simulink model "beetleBotFull"  (R2016a)
settings: Solver=VariableStepAuto  StartTime=0.0  StopTime=simTime  MaxStep=0.001  RelTol=1e-3
model workspace: external: MAT-File C:\Users\dpied\Documents\Carnegie Mellon\2nd Semester\KDC\Project\Segway_Simulation\beetleBot_DataFile.mat (data not in the file)
undefined symbols (not defined in the file or in its folder): Ddecouple, ground_y, Kbalance, Kflight, Kturn, motorSaturation, smiData, state_desired, table, table_height, table_y, X, Y, Z
libraries: sm_lib x149, nesl_utility x15, Contact_Forces_Lib x8, simulink x2
(part 1 of 4)
settings Model: Creator=dpied  LastModifiedBy=dpied
settings GRTTargetCC: GeneratePreprocessorConditionals=Use local settings

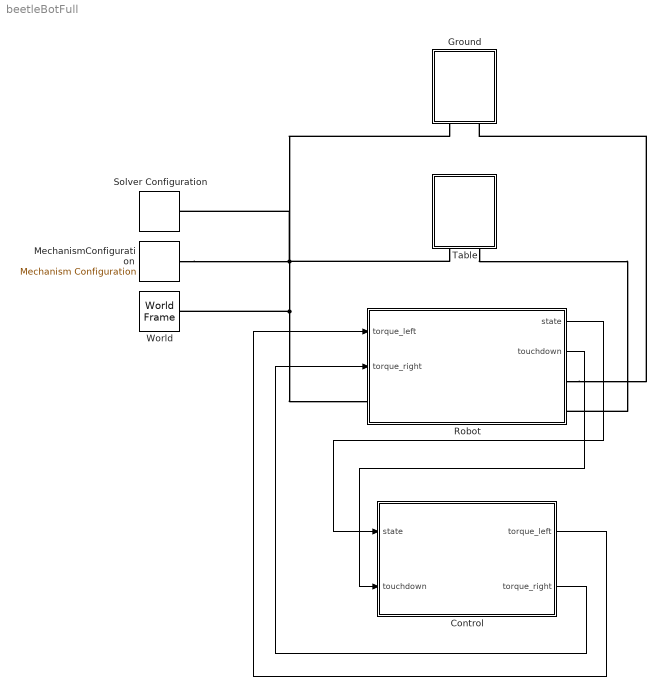
== system beetleBotFull ==
  Control : Subsystem
  Ground : Subsystem
  MechanismConfiguration : sm_lib/Utilities/Mechanism Configuration  UniformGravity=Constant  GravityVector=[0 0 -9.81]  GravityUnits=m/s^2  LinearizationDelta=0.001
  Robot : Subsystem
  Solver Configuration : nesl_utility/Solver Configuration  PhysicalDomain=network_engine_domain  SubClassName=solver  LeftPortType=input  RightPortType=generic  Accelerate=off  Tones=[]  Harmonics=[]  SimulateNoise=off  Profile=off  UseLocalSampling=off  EnableSwitchedLinearOptims=on  FrequencyDomain=off  UseCCode=off  RelTol=0.001  AbsTol=1e-06  MinStep=1e-09  ToWorkspace=off  RevertToSquareIcSolve=off  NumHomotopyIterations=100  PhasorMode=off  PhasorModeNumHarmonics=1  OverrideAbsTol=off  DoDC=off  ResidualTolerance=1e-09  UseLocalSolver=off  LocalSolverChoice=NE_BACKWARD_EULER_ADVANCER  LocalSolverSampleTime=0.001  DoFixedCost=off  MaxNonlinIter=3  MaxModeIter=2  LinearAlgebra=Sparse  DelaysMemoryBudget=1024  AutomaticFiltering=on  FilteringTimeConstant=0.001
  Table : Subsystem
  World : sm_lib/Frames and Transforms/World Frame
  wires:
  Robot/1(state) -> Control/1(state)
  Control/1(torque_left) -> Robot/1(torque_left)
  Control/2(torque_right) -> Robot/2(torque_right)
  Robot/2(touchdown) -> Control/2(touchdown)
  connections:
  MechanismConfiguration/RConn1 -- Robot/LConn1 -- World/RConn1 -- Table/LConn1 -- Ground/LConn1 -- Solver Configuration/RConn1
  Robot/RConn1 -- Ground/LConn2
  Table/LConn2 -- Robot/RConn2

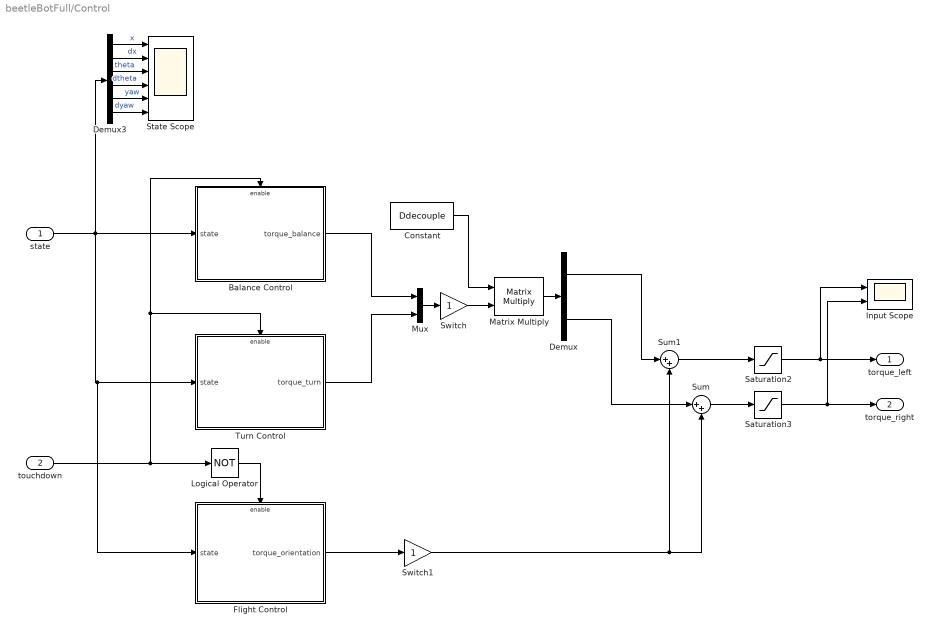
== system beetleBotFull/Control ==
  state : Inport
  touchdown : Inport  Port=2
  Balance Control : Subsystem
  Constant : Constant  Value=Ddecouple
  Demux : Demux  Outputs=2
  Demux3 : Demux  Outputs=6
  Flight Control : Subsystem
  Input Scope : Scope  NumInputPorts=2
  Logical Operator : Logic  Operator=NOT  AllPortsSameDT=off  OutDataTypeStr=boolean
  Matrix Multiply : Product  Multiplication=Matrix(*)
  Mux : Mux  Inputs=2
  Saturation2 : Saturate  UpperLimit=motorSaturation  LowerLimit=-motorSaturation
  Saturation3 : Saturate  UpperLimit=motorSaturation  LowerLimit=-motorSaturation
  State Scope : Scope  NumInputPorts=6
  Sum : Sum  Inputs=|++
  Sum1 : Sum  Inputs=|++
  Switch : Gain
  Switch1 : Gain
  Turn Control : Subsystem
  torque_left : Outport
  torque_right : Outport  Port=2
  wires:
  state/1 -> Flight Control/1(state), Turn Control/1(state), Balance Control/1(state), Demux3/1
  Saturation2/1 -> Input Scope/1, torque_left/1
  Saturation3/1 -> Input Scope/2, torque_right/1
  Demux3/1 -> State Scope/1  "x"
  Demux3/2 -> State Scope/2  "dx"
  touchdown/1 -> Balance Control/Enable, Turn Control/Enable, Logical Operator/1
  Demux3/3 -> State Scope/3  "theta"
  Demux3/4 -> State Scope/4  "dtheta"
  Demux3/5 -> State Scope/5  "yaw"
  Demux3/6 -> State Scope/6  "dyaw"
  Balance Control/1(torque_balance) -> Mux/1
  Turn Control/1(torque_turn) -> Mux/2
  Mux/1 -> Switch/1
  Constant/1 -> Matrix Multiply/1
  Matrix Multiply/1 -> Demux/1
  Switch/1 -> Matrix Multiply/2
  Logical Operator/1 -> Flight Control/Enable
  Sum/1 -> Saturation3/1
  Demux/2 -> Sum/1
  Sum1/1 -> Saturation2/1
  Demux/1 -> Sum1/1
  Flight Control/1(torque_orientation) -> Switch1/1
  Switch1/1 -> Sum1/2, Sum/2

== system beetleBotFull/Ground ==
  Constant : Constant  Value=0
  Constant1 : Constant  Value=0
  Ground : Subsystem  Tag=CustomStyle
  Simulink-PS Converter : nesl_utility/Simulink-PS Converter  PhysicalDomain=network_engine_domain  SubClassName=ps_input  LeftPortType=input  RightPortType=output  PseudoPeriodic=off  Frequencies=[]  NoiseDistribution=none  NoiseParameters=[]  Unit=1  AffineConversion=off  InputFiltering=off  SimscapeFilterOrder=1  InputFilterTimeConstant=0.001  UdotUserProvided=1
  Simulink-PS Converter1 : nesl_utility/Simulink-PS Converter  PhysicalDomain=network_engine_domain  SubClassName=ps_input  LeftPortType=input  RightPortType=output  PseudoPeriodic=off  Frequencies=[]  NoiseDistribution=none  NoiseParameters=[]  Unit=1  AffineConversion=off  InputFiltering=off  SimscapeFilterOrder=1  InputFilterTimeConstant=0.001  UdotUserProvided=1
  Universal Joint : sm_lib/Joints/Universal Joint  SenseConstraintForce=off  SenseConstraintForceX=off  SenseConstraintForceY=off  SenseConstraintForceZ=off  SenseConstraintTorque=off  SenseConstraintTorqueX=off  SenseConstraintTorqueY=off  SenseConstraintTorqueZ=off  SenseTotalForce=off  SenseTotalForceX=off  SenseTotalForceY=off  SenseTotalForceZ=off  SenseTotalTorque=off  SenseTotalTorqueX=off  SenseTotalTorqueY=off  SenseTotalTorqueZ=off  CompositeWrenchDir=FollowerOnBase  CompositeWrenchFrame=BaseFrame  RxEquilibriumPosition=0  RxEquilibriumPositionUnits=deg  RxSpringStiffness=0  RxSpringStiffnessUnits=N*m/deg  RxDampingCoefficient=0  RxDampingCoefficientUnits=N*m/(deg/s)  RxTorqueActuationMode=ComputedTorque  RxMotionActuationMode=InputMotion  RxSensePosition=off  RxSenseVelocity=off  RxSenseAcceleration=off  RxSenseTorqueForce=off  RxPositionTargetSpecify=off  RxPositionTargetPriority=High  RxPositionTargetValue=0  RxPositionTargetValueUnits=deg  RxVelocityTargetSpecify=off  RxVelocityTargetPriority=High  RxVelocityTargetValue=0  RxVelocityTargetValueUnits=deg/s  RyEquilibriumPosition=0  RyEquilibriumPositionUnits=deg  RySpringStiffness=0  RySpringStiffnessUnits=N*m/deg  RyDampingCoefficient=0  RyDampingCoefficientUnits=N*m/(deg/s)  RyTorqueActuationMode=ComputedTorque  RyMotionActuationMode=InputMotion  RySensePosition=off  RySenseVelocity=off  RySenseAcceleration=off  RySenseTorqueForce=off  RyPositionTargetSpecify=off  RyPositionTargetPriority=High  RyPositionTargetValue=0  RyPositionTargetValueUnits=deg  RyVelocityTargetSpecify=off  RyVelocityTargetPriority=High  RyVelocityTargetValue=0  RyVelocityTargetValueUnits=deg/s
  worldFrame : PMIOPort  Port=1  Side=Left
  groundFrame : PMIOPort  Port=2  Side=Left
  wires:
  Constant/1 -> Simulink-PS Converter/1
  Constant1/1 -> Simulink-PS Converter1/1
  connections:
  Ground/LConn1 -- Universal Joint/RConn1
  Simulink-PS Converter/RConn1 -- Universal Joint/LConn2
  Simulink-PS Converter1/RConn1 -- Universal Joint/LConn3
  groundFrame/RConn1 -- Ground/RConn1
  Universal Joint/LConn1 -- worldFrame/RConn1

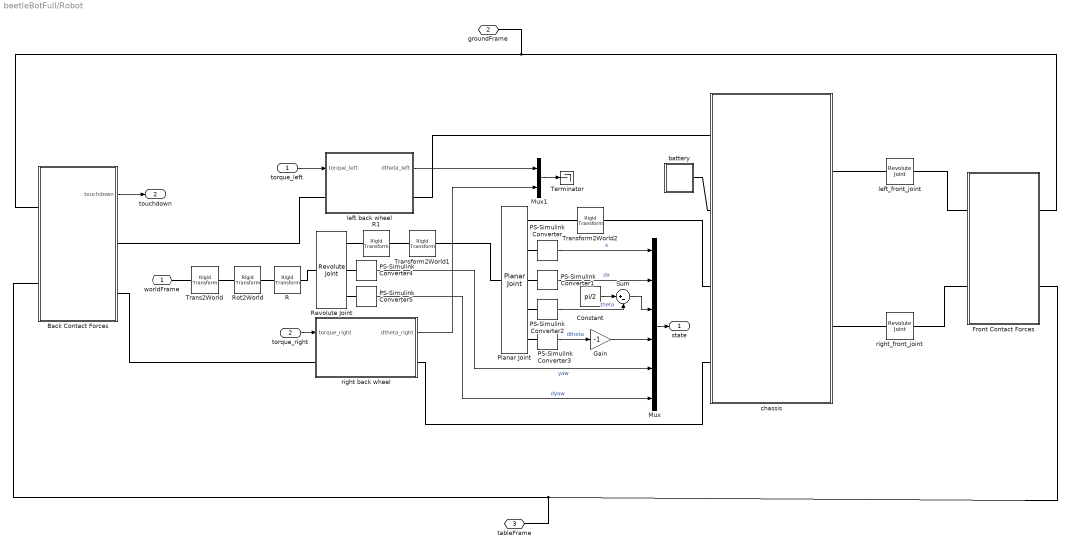
== system beetleBotFull/Robot ==
  torque_left : Inport
  torque_right : Inport  Port=2
  Back Contact Forces : Subsystem
  Constant : Constant  Value=pi/2
  Front Contact Forces : Subsystem
  Gain : Gain  Gain=-1
  Mux : Mux  Inputs=6
  Mux1 : Mux  Inputs=2
  PS-Simulink Converter{,1..5} (6 alike) : nesl_utility/PS-Simulink Converter  PhysicalDomain=network_engine_domain  SubClassName=ps_output  LeftPortType=input  RightPortType=output  PseudoPeriodic=off  Frequencies=[]  Unit=1  AffineConversion=off
  Planar Joint : sm_lib/Joints/Planar Joint  SenseConstraintForce=off  SenseConstraintForceX=off  SenseConstraintForceY=off  SenseConstraintForceZ=off  SenseConstraintTorque=off  SenseConstraintTorqueX=off  SenseConstraintTorqueY=off  SenseConstraintTorqueZ=off  SenseTotalForce=off  SenseTotalForceX=off  SenseTotalForceY=off  SenseTotalForceZ=off  SenseTotalTorque=off  SenseTotalTorqueX=off  SenseTotalTorqueY=off  SenseTotalTorqueZ=off  CompositeWrenchDir=FollowerOnBase  CompositeWrenchFrame=BaseFrame  PxEquilibriumPosition=0  PxEquilibriumPositionUnits=m  PxSpringStiffness=0  PxSpringStiffnessUnits=N/m  PxDampingCoefficient=0  PxDampingCoefficientUnits=N/(m/s)  PxTorqueActuationMode=NoTorque  PxMotionActuationMode=ComputedMotion  PxSensePosition=on  PxSenseVelocity=on  PxSenseAcceleration=off  PxSenseTorqueForce=off  PxPositionTargetSpecify=on  PxPositionTargetPriority=High  PxPositionTargetValue=x_initial  PxPositionTargetValueUnits=m  PxVelocityTargetSpecify=on  PxVelocityTargetPriority=High  PxVelocityTargetValue=dx_initial  PxVelocityTargetValueUnits=m/s  PyEquilibriumPosition=0  PyEquilibriumPositionUnits=m  PySpringStiffness=0  PySpringStiffnessUnits=N/m  PyDampingCoefficient=0  PyDampingCoefficientUnits=N/(m/s)  PyTorqueActuationMode=NoTorque  PyMotionActuationMode=ComputedMotion  PySensePosition=off  PySenseVelocity=off  PySenseAcceleration=off  PySenseTorqueForce=off  PyPositionTargetSpecify=on  PyPositionTargetPriority=High  PyPositionTargetValue=initial_height  PyPositionTargetValueUnits=m  PyVelocityTargetSpecify=off  PyVelocityTargetPriority=High  PyVelocityTargetValue=0  PyVelocityTargetValueUnits=m/s  RzEquilibriumPosition=0  RzEquilibriumPositionUnits=deg  RzSpringStiffness=0  RzSpringStiffnessUnits=N*m/deg  RzDampingCoefficient=0  RzDampingCoefficientUnits=N*m/(deg/s)  RzTorqueActuationMode=NoTorque  RzMotionActuationMode=ComputedMotion  RzSensePosition=on  RzSenseVelocity=on  RzSenseAcceleration=off  RzSenseTorqueForce=off  RzPositionTargetSpecify=on  RzPositionTargetPriority=High  RzPositionTargetValue=theta_initial  RzPositionTargetValueUnits=deg  RzVelocityTargetSpecify=off  RzVelocityTargetPriority=High  RzVelocityTargetValue=0  RzVelocityTargetValueUnits=deg/s
  R : sm_lib/Frames and Transforms/Rigid Transform  TranslationMethod=None  TranslationLengthUnit=mm  TranslationStandardAxis=+Z  TranslationStandardOffset=0  TranslationCartesianOffset=smiData.RigidTransform(51).translation  TranslationROffset=0  TranslationROffsetUnits=m  TranslationZOffset=0  TranslationZOffsetUnits=m  TranslationThetaOffset=0  TranslationThetaOffsetUnits=deg  RotationMethod=StandardAxis  RotationAngleUnits=rad  RotationStandardAxis=+X  RotationAngle=-pi/2  RotationArbitraryAxis=smiData.RigidTransform(51).axis  FollAlignAxisA=+X  BaseAlignAxisA=+Y  FollAlignAxisB=+Y  BaseAlignAxisB=+Z  RotationSequenceAxes=FollowerAxes  RotationSequence=XYX  RotationSequenceAngles=[0 0 0]  RotationSequenceAnglesUnits=deg  RotationMatrix=[1 0 0; 0 1 0; 0 0 1]
  R1 : sm_lib/Frames and Transforms/Rigid Transform  TranslationMethod=None  TranslationLengthUnit=mm  TranslationStandardAxis=+Z  TranslationStandardOffset=0  TranslationCartesianOffset=smiData.RigidTransform(51).translation  TranslationROffset=0  TranslationROffsetUnits=m  TranslationZOffset=0  TranslationZOffsetUnits=m  TranslationThetaOffset=0  TranslationThetaOffsetUnits=deg  RotationMethod=StandardAxis  RotationAngleUnits=rad  RotationStandardAxis=+X  RotationAngle=pi/2  RotationArbitraryAxis=smiData.RigidTransform(51).axis  FollAlignAxisA=+X  BaseAlignAxisA=+Y  FollAlignAxisB=+Y  BaseAlignAxisB=+Z  RotationSequenceAxes=FollowerAxes  RotationSequence=XYX  RotationSequenceAngles=[0 0 0]  RotationSequenceAnglesUnits=deg  RotationMatrix=[1 0 0; 0 1 0; 0 0 1]
  Revolute Joint : sm_lib/Joints/Revolute Joint  SenseConstraintForce=off  SenseConstraintForceX=off  SenseConstraintForceY=off  SenseConstraintForceZ=off  SenseConstraintTorque=off  SenseConstraintTorqueX=off  SenseConstraintTorqueY=off  SenseConstraintTorqueZ=off  SenseTotalForce=off  SenseTotalForceX=off  SenseTotalForceY=off  SenseTotalForceZ=off  SenseTotalTorque=off  SenseTotalTorqueX=off  SenseTotalTorqueY=off  SenseTotalTorqueZ=off  CompositeWrenchDir=FollowerOnBase  CompositeWrenchFrame=BaseFrame  EquilibriumPosition=0  EquilibriumPositionUnits=deg  SpringStiffness=0  SpringStiffnessUnits=N*m/deg  DampingCoefficient=0  DampingCoefficientUnits=N*m/(deg/s)  TorqueActuationMode=NoTorque  MotionActuationMode=ComputedMotion  SensePosition=on  SenseVelocity=on  SenseAcceleration=off  SenseTorqueForce=off  PositionTargetSpecify=off  PositionTargetPriority=High  PositionTargetValue=0  PositionTargetValueUnits=deg  VelocityTargetSpecify=off  VelocityTargetPriority=High  VelocityTargetValue=0  VelocityTargetValueUnits=deg/s
  Rot2World : sm_lib/Frames and Transforms/Rigid Transform  TranslationMethod=None  TranslationLengthUnit=mm  TranslationStandardAxis=+Z  TranslationStandardOffset=0  TranslationCartesianOffset=smiData.RigidTransform(51).translation  TranslationROffset=0  TranslationROffsetUnits=m  TranslationZOffset=0  TranslationZOffsetUnits=m  TranslationThetaOffset=0  TranslationThetaOffsetUnits=deg  RotationMethod=StandardAxis  RotationAngleUnits=rad  RotationStandardAxis=+X  RotationAngle=pi/2  RotationArbitraryAxis=smiData.RigidTransform(51).axis  FollAlignAxisA=+X  BaseAlignAxisA=+Y  FollAlignAxisB=+Y  BaseAlignAxisB=+Z  RotationSequenceAxes=FollowerAxes  RotationSequence=XYX  RotationSequenceAngles=[0 0 0]  RotationSequenceAnglesUnits=deg  RotationMatrix=[1 0 0; 0 1 0; 0 0 1]
  Sum : Sum  Inputs=|+-
  Terminator : Terminator
  Trans2World : sm_lib/Frames and Transforms/Rigid Transform  TranslationMethod=Cartesian  TranslationLengthUnit=m  TranslationStandardAxis=+Z  TranslationStandardOffset=0  TranslationCartesianOffset=[0 0 0.118]  TranslationROffset=0  TranslationROffsetUnits=m  TranslationZOffset=0  TranslationZOffsetUnits=m  TranslationThetaOffset=0  TranslationThetaOffsetUnits=deg  RotationMethod=None  RotationAngleUnits=rad  RotationStandardAxis=+X  RotationAngle=pi/2  RotationArbitraryAxis=smiData.RigidTransform(51).axis  FollAlignAxisA=+X  BaseAlignAxisA=+Y  FollAlignAxisB=+Y  BaseAlignAxisB=+Z  RotationSequenceAxes=FollowerAxes  RotationSequence=XYX  RotationSequenceAngles=[0 0 0]  RotationSequenceAnglesUnits=deg  RotationMatrix=[1 0 0; 0 1 0; 0 0 1]
  Transform2World1 : sm_lib/Frames and Transforms/Rigid Transform  TranslationMethod=None  TranslationLengthUnit=mm  TranslationStandardAxis=+Z  TranslationStandardOffset=0  TranslationCartesianOffset=smiData.RigidTransform(51).translation  TranslationROffset=0  TranslationROffsetUnits=m  TranslationZOffset=0  TranslationZOffsetUnits=m  TranslationThetaOffset=0  TranslationThetaOffsetUnits=deg  RotationMethod=StandardAxis  RotationAngleUnits=rad  RotationStandardAxis=+Y  RotationAngle=-pi/2  RotationArbitraryAxis=smiData.RigidTransform(51).axis  FollAlignAxisA=+X  BaseAlignAxisA=+Y  FollAlignAxisB=+Y  BaseAlignAxisB=+Z  RotationSequenceAxes=FollowerAxes  RotationSequence=XYX  RotationSequenceAngles=[0 0 0]  RotationSequenceAnglesUnits=deg  RotationMatrix=[1 0 0; 0 1 0; 0 0 1]
  Transform2World2 : sm_lib/Frames and Transforms/Rigid Transform  TranslationMethod=None  TranslationLengthUnit=mm  TranslationStandardAxis=+Z  TranslationStandardOffset=0  TranslationCartesianOffset=smiData.RigidTransform(51).translation  TranslationROffset=0  TranslationROffsetUnits=m  TranslationZOffset=0  TranslationZOffsetUnits=m  TranslationThetaOffset=0  TranslationThetaOffsetUnits=deg  RotationMethod=StandardAxis  RotationAngleUnits=rad  RotationStandardAxis=+Y  RotationAngle=pi/2  RotationArbitraryAxis=smiData.RigidTransform(51).axis  FollAlignAxisA=+X  BaseAlignAxisA=+Y  FollAlignAxisB=+Y  BaseAlignAxisB=+Z  RotationSequenceAxes=FollowerAxes  RotationSequence=XYX  RotationSequenceAngles=[0 0 0]  RotationSequenceAnglesUnits=deg  RotationMatrix=[1 0 0; 0 1 0; 0 0 1]
  battery : Subsystem
  chassis : Subsystem
  left back wheel : Subsystem
  left_front_joint : sm_lib/Joints/Revolute Joint  SenseConstraintForce=off  SenseConstraintForceX=off  SenseConstraintForceY=off  SenseConstraintForceZ=off  SenseConstraintTorque=off  SenseConstraintTorqueX=off  SenseConstraintTorqueY=off  SenseConstraintTorqueZ=off  SenseTotalForce=off  SenseTotalForceX=off  SenseTotalForceY=off  SenseTotalForceZ=off  SenseTotalTorque=off  SenseTotalTorqueX=off  SenseTotalTorqueY=off  SenseTotalTorqueZ=off  CompositeWrenchDir=FollowerOnBase  CompositeWrenchFrame=BaseFrame  EquilibriumPosition=0  EquilibriumPositionUnits=rad  SpringStiffness=0  SpringStiffnessUnits=m*N/rad  DampingCoefficient=0  DampingCoefficientUnits=m*s*N/rad  TorqueActuationMode=NoTorque  MotionActuationMode=ComputedMotion  SensePosition=off  SenseVelocity=off  SenseAcceleration=off  SenseTorqueForce=off  PositionTargetSpecify=on  PositionTargetPriority=Low  PositionTargetValue=0  PositionTargetValueUnits=deg  VelocityTargetSpecify=off  VelocityTargetPriority=High  VelocityTargetValue=0  VelocityTargetValueUnits=deg/s
  right back wheel : Subsystem
  right_front_joint : sm_lib/Joints/Revolute Joint  SenseConstraintForce=off  SenseConstraintForceX=off  SenseConstraintForceY=off  SenseConstraintForceZ=off  SenseConstraintTorque=off  SenseConstraintTorqueX=off  SenseConstraintTorqueY=off  SenseConstraintTorqueZ=off  SenseTotalForce=off  SenseTotalForceX=off  SenseTotalForceY=off  SenseTotalForceZ=off  SenseTotalTorque=off  SenseTotalTorqueX=off  SenseTotalTorqueY=off  SenseTotalTorqueZ=off  CompositeWrenchDir=FollowerOnBase  CompositeWrenchFrame=BaseFrame  EquilibriumPosition=0  EquilibriumPositionUnits=rad  SpringStiffness=0  SpringStiffnessUnits=m*N/rad  DampingCoefficient=0  DampingCoefficientUnits=m*s*N/rad  TorqueActuationMode=NoTorque  MotionActuationMode=ComputedMotion  SensePosition=off  SenseVelocity=off  SenseAcceleration=off  SenseTorqueForce=off  PositionTargetSpecify=on  PositionTargetPriority=Low  PositionTargetValue=0  PositionTargetValueUnits=deg  VelocityTargetSpecify=off  VelocityTargetPriority=High  VelocityTargetValue=0  VelocityTargetValueUnits=deg/s
  worldFrame : PMIOPort  Port=1  Side=Left
  groundFrame : PMIOPort  Port=2  Side=Right
  tableFrame : PMIOPort  Port=3  Side=Right
  state : Outport
  touchdown : Outport  Port=2
  wires:
  torque_left/1 -> left back wheel/1(torque_left)
  Mux/1 -> state/1
  Mux1/1 -> Terminator/1
  left back wheel/1(dtheta_left) -> Mux1/1
  right back wheel/1(dtheta_right) -> Mux1/2
  torque_right/1 -> right back wheel/1(torque_right)
  Back Contact Forces/1(touchdown) -> touchdown/1
  PS-Simulink Converter2/1 -> Sum/2  "theta"
  PS-Simulink Converter3/1 -> Gain/1  "dtheta"
  Sum/1 -> Mux/3
  Constant/1 -> Sum/1
  PS-Simulink Converter/1 -> Mux/1  "x"
  PS-Simulink Converter1/1 -> Mux/2  "dx"
  Gain/1 -> Mux/4
  PS-Simulink Converter4/1 -> Mux/5  "yaw"
  PS-Simulink Converter5/1 -> Mux/6  "dyaw"
  connections:
  Trans2World/RConn1 -- Rot2World/LConn1
  battery/LConn1 -- chassis/LConn2
  worldFrame/RConn1 -- Trans2World/LConn1
  chassis/LConn1 -- left back wheel/RConn1
  chassis/LConn4 -- right back wheel/RConn1
  Transform2World2/LConn1 -- Planar Joint/RConn1
  left_front_joint/LConn1 -- chassis/RConn1
  right_front_joint/LConn1 -- chassis/RConn2
  Transform2World2/RConn1 -- chassis/LConn3
  R/LConn1 -- Rot2World/RConn1
  groundFrame/RConn1 -- Back Contact Forces/LConn1 -- Front Contact Forces/RConn1
  Front Contact Forces/LConn1 -- left_front_joint/RConn1
  Front Contact Forces/LConn2 -- right_front_joint/RConn1
  Back Contact Forces/RConn1 -- left back wheel/LConn1
  Back Contact Forces/RConn2 -- right back wheel/LConn1
  PS-Simulink Converter/LConn1 -- Planar Joint/RConn2
  PS-Simulink Converter1/LConn1 -- Planar Joint/RConn3
  Planar Joint/RConn4 -- PS-Simulink Converter2/LConn1
  Planar Joint/RConn5 -- PS-Simulink Converter3/LConn1
  Transform2World1/RConn1 -- Planar Joint/LConn1
  Transform2World1/LConn1 -- R1/RConn1
  Revolute Joint/LConn1 -- R/RConn1
  R1/LConn1 -- Revolute Joint/RConn1
  PS-Simulink Converter4/LConn1 -- Revolute Joint/RConn2
  PS-Simulink Converter5/LConn1 -- Revolute Joint/RConn3
  tableFrame/RConn1 -- Back Contact Forces/LConn2 -- Front Contact Forces/RConn2

== system beetleBotFull/Table ==
  Constant : Constant  Value=0
  Constant1 : Constant  Value=0
  Simulink-PS Converter : nesl_utility/Simulink-PS Converter  PhysicalDomain=network_engine_domain  SubClassName=ps_input  LeftPortType=input  RightPortType=output  PseudoPeriodic=off  Frequencies=[]  NoiseDistribution=none  NoiseParameters=[]  Unit=1  AffineConversion=off  InputFiltering=off  SimscapeFilterOrder=1  InputFilterTimeConstant=0.001  UdotUserProvided=1
  Simulink-PS Converter1 : nesl_utility/Simulink-PS Converter  PhysicalDomain=network_engine_domain  SubClassName=ps_input  LeftPortType=input  RightPortType=output  PseudoPeriodic=off  Frequencies=[]  NoiseDistribution=none  NoiseParameters=[]  Unit=1  AffineConversion=off  InputFiltering=off  SimscapeFilterOrder=1  InputFilterTimeConstant=0.001  UdotUserProvided=1
  Table : Subsystem  Tag=CustomStyle
  Universal Joint : sm_lib/Joints/Universal Joint  SenseConstraintForce=off  SenseConstraintForceX=off  SenseConstraintForceY=off  SenseConstraintForceZ=off  SenseConstraintTorque=off  SenseConstraintTorqueX=off  SenseConstraintTorqueY=off  SenseConstraintTorqueZ=off  SenseTotalForce=off  SenseTotalForceX=off  SenseTotalForceY=off  SenseTotalForceZ=off  SenseTotalTorque=off  SenseTotalTorqueX=off  SenseTotalTorqueY=off  SenseTotalTorqueZ=off  CompositeWrenchDir=FollowerOnBase  CompositeWrenchFrame=BaseFrame  RxEquilibriumPosition=0  RxEquilibriumPositionUnits=deg  RxSpringStiffness=0  RxSpringStiffnessUnits=N*m/deg  RxDampingCoefficient=0  RxDampingCoefficientUnits=N*m/(deg/s)  RxTorqueActuationMode=ComputedTorque  RxMotionActuationMode=InputMotion  RxSensePosition=off  RxSenseVelocity=off  RxSenseAcceleration=off  RxSenseTorqueForce=off  RxPositionTargetSpecify=off  RxPositionTargetPriority=High  RxPositionTargetValue=0  RxPositionTargetValueUnits=deg  RxVelocityTargetSpecify=off  RxVelocityTargetPriority=High  RxVelocityTargetValue=0  RxVelocityTargetValueUnits=deg/s  RyEquilibriumPosition=0  RyEquilibriumPositionUnits=deg  RySpringStiffness=0  RySpringStiffnessUnits=N*m/deg  RyDampingCoefficient=0  RyDampingCoefficientUnits=N*m/(deg/s)  RyTorqueActuationMode=ComputedTorque  RyMotionActuationMode=InputMotion  RySensePosition=off  RySenseVelocity=off  RySenseAcceleration=off  RySenseTorqueForce=off  RyPositionTargetSpecify=off  RyPositionTargetPriority=High  RyPositionTargetValue=0  RyPositionTargetValueUnits=deg  RyVelocityTargetSpecify=off  RyVelocityTargetPriority=High  RyVelocityTargetValue=0  RyVelocityTargetValueUnits=deg/s
  worldFrame : PMIOPort  Port=1  Side=Left
  tableFrame : PMIOPort  Port=2  Side=Left
  wires:
  Constant/1 -> Simulink-PS Converter/1
  Constant1/1 -> Simulink-PS Converter1/1
  connections:
  Table/LConn1 -- Universal Joint/RConn1
  Simulink-PS Converter/RConn1 -- Universal Joint/LConn2
  Simulink-PS Converter1/RConn1 -- Universal Joint/LConn3
  tableFrame/RConn1 -- Table/RConn1
  Universal Joint/LConn1 -- worldFrame/RConn1

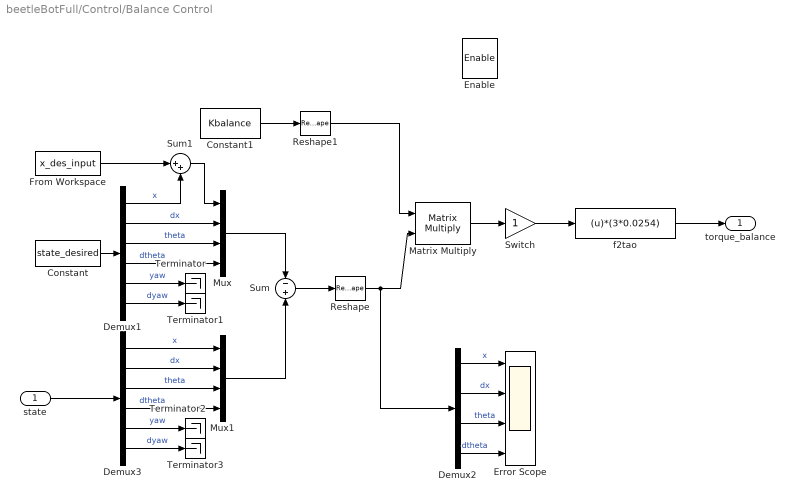
== system beetleBotFull/Control/Balance Control ==
  state : Inport
  Enable : EnablePort
  Constant : Constant  Value=state_desired
  Constant1 : Constant  Value=Kbalance
  Demux1 : Demux  Outputs=6
  Demux2 : Demux
  Demux3 : Demux  Outputs=6
  Error Scope : Scope  NumInputPorts=4
  From Workspace : FromWorkspace  VariableName=x_des_input  SampleTime=0
  Matrix Multiply : Product  Multiplication=Matrix(*)
  Mux : Mux
  Mux1 : Mux
  Reshape : Reshape  OutputDimensionality=Column vector (2-D)
  Reshape1 : Reshape  OutputDimensionality=Row vector (2-D)
  Sum : Sum  Inputs=-+
  Sum1 : Sum  Inputs=|++
  Switch : Gain
  Terminator{,1..3} (4 alike) : Terminator
  f2tao : Fcn  Expr=(u)*(3*0.0254)
  torque_balance : Outport  OutputWhenDisabled=reset  InitialOutput=0
  wires:
  Matrix Multiply/1 -> Switch/1
  Constant1/1 -> Reshape1/1
  Sum/1 -> Reshape/1
  Reshape1/1 -> Matrix Multiply/1
  Switch/1 -> f2tao/1
  Constant/1 -> Demux1/1
  Mux/1 -> Sum/1
  Demux1/1 -> Sum1/2  "x"
  Sum1/1 -> Mux/1
  From Workspace/1 -> Sum1/1
  Demux1/2 -> Mux/2  "dx"
  Demux1/3 -> Mux/3  "theta"
  Demux1/4 -> Mux/4  "dtheta"
  Demux2/1 -> Error Scope/1  "x"
  Demux2/2 -> Error Scope/2  "dx"
  Demux2/3 -> Error Scope/3  "theta"
  Demux2/4 -> Error Scope/4  "dtheta"
  Demux1/5 -> Terminator/1  "yaw"
  Demux1/6 -> Terminator1/1  "dyaw"
  Mux1/1 -> Sum/2
  Demux3/2 -> Mux1/2  "dx"
  Demux3/3 -> Mux1/3  "theta"
  Demux3/4 -> Mux1/4  "dtheta"
  Demux3/5 -> Terminator2/1  "yaw"
  Demux3/6 -> Terminator3/1  "dyaw"
  Demux3/1 -> Mux1/1  "x"
  state/1 -> Demux3/1
  f2tao/1 -> torque_balance/1
  Reshape/1 -> Demux2/1, Matrix Multiply/2

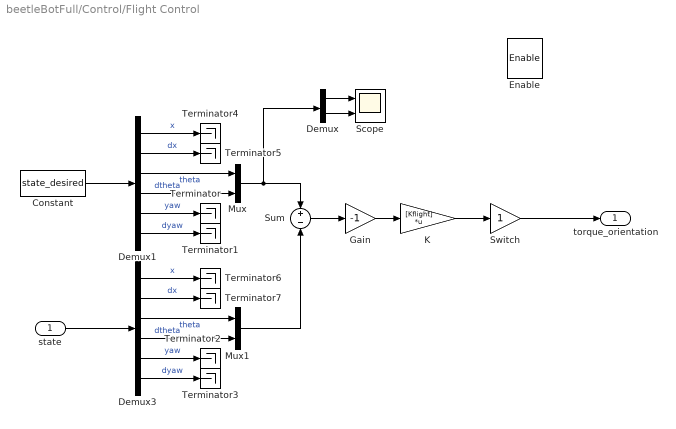
== system beetleBotFull/Control/Flight Control ==
  state : Inport
  Enable : EnablePort
  Constant : Constant  Value=state_desired
  Demux : Demux  Outputs=2
  Demux1 : Demux  Outputs=6
  Demux3 : Demux  Outputs=6
  Gain : Gain  Gain=-1
  K : Gain  Gain=[Kflight]  Multiplication=Matrix(K*u)
  Mux : Mux  Inputs=2
  Mux1 : Mux  Inputs=2
  Scope : Scope  NumInputPorts=2
  Sum : Sum  Inputs=+-
  Switch : Gain
  Terminator{,1..7} (8 alike) : Terminator
  torque_orientation : Outport  OutputWhenDisabled=reset  InitialOutput=0
  wires:
  K/1 -> Switch/1
  Switch/1 -> torque_orientation/1
  Demux/1 -> Scope/1
  Demux/2 -> Scope/2
  Sum/1 -> Gain/1
  Gain/1 -> K/1
  Constant/1 -> Demux1/1
  Mux/1 -> Demux/1, Sum/1
  Demux1/3 -> Mux/1  "theta"
  Demux1/4 -> Mux/2  "dtheta"
  Demux1/5 -> Terminator/1  "yaw"
  Demux1/6 -> Terminator1/1  "dyaw"
  Mux1/1 -> Sum/2
  Demux3/3 -> Mux1/1  "theta"
  Demux3/4 -> Mux1/2  "dtheta"
  Demux3/5 -> Terminator2/1  "yaw"
  Demux3/6 -> Terminator3/1  "dyaw"
  state/1 -> Demux3/1
  Demux1/1 -> Terminator4/1  "x"
  Demux1/2 -> Terminator5/1  "dx"
  Demux3/1 -> Terminator6/1  "x"
  Demux3/2 -> Terminator7/1  "dx"

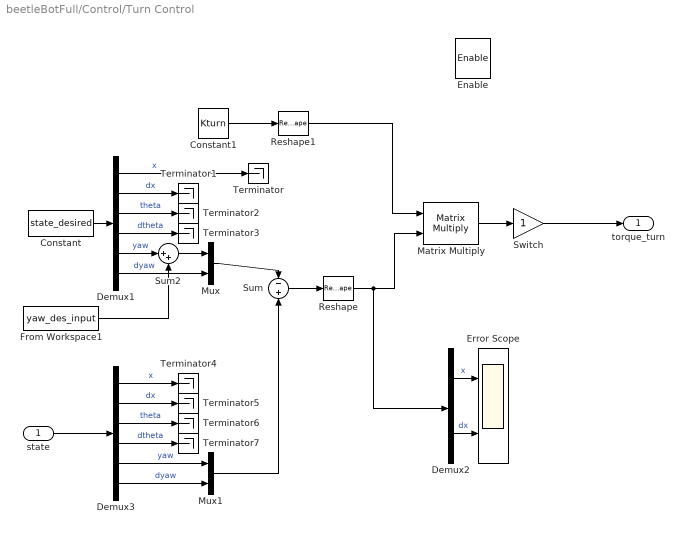
== system beetleBotFull/Control/Turn Control ==
  state : Inport
  Enable : EnablePort
  Constant : Constant  Value=state_desired
  Constant1 : Constant  Value=Kturn
  Demux1 : Demux  Outputs=6
  Demux2 : Demux  Outputs=2
  Demux3 : Demux  Outputs=6
  Error Scope : Scope  NumInputPorts=2
  From Workspace1 : FromWorkspace  VariableName=yaw_des_input  SampleTime=0
  Matrix Multiply : Product  Multiplication=Matrix(*)
  Mux : Mux  Inputs=2
  Mux1 : Mux  Inputs=2
  Reshape : Reshape  OutputDimensionality=Column vector (2-D)
  Reshape1 : Reshape  OutputDimensionality=Row vector (2-D)
  Sum : Sum  Inputs=-+
  Sum2 : Sum  Inputs=|++
  Switch : Gain
  Terminator{,1..7} (8 alike) : Terminator
  torque_turn : Outport  OutputWhenDisabled=reset  InitialOutput=0
  wires:
  Matrix Multiply/1 -> Switch/1
  Constant1/1 -> Reshape1/1
  Sum/1 -> Reshape/1
  Reshape1/1 -> Matrix Multiply/1
  Switch/1 -> torque_turn/1
  Constant/1 -> Demux1/1
  Mux/1 -> Sum/1
  Demux1/6 -> Mux/2  "dyaw"
  Demux1/5 -> Sum2/1  "yaw"
  Sum2/1 -> Mux/1
  From Workspace1/1 -> Sum2/2
  Demux1/1 -> Terminator/1  "x"
  Demux1/2 -> Terminator1/1  "dx"
  Demux1/3 -> Terminator2/1  "theta"
  Demux1/4 -> Terminator3/1  "dtheta"
  state/1 -> Demux3/1
  Demux3/6 -> Mux1/2  "dyaw"
  Demux3/5 -> Mux1/1  "yaw"
  Demux3/1 -> Terminator4/1  "x"
  Demux3/2 -> Terminator5/1  "dx"
  Demux3/3 -> Terminator6/1  "theta"
  Demux3/4 -> Terminator7/1  "dtheta"
  Mux1/1 -> Sum/2
  Demux2/1 -> Error Scope/1  "x"
  Demux2/2 -> Error Scope/2  "dx"
  Reshape/1 -> Demux2/1, Matrix Multiply/2

== system beetleBotFull/Ground/Ground ==
  Solid : sm_lib/Body Elements/Solid  InertiaType=CalculateFromGeometry  Mass=1  MassUnits=kg  CenterOfMass=[0 0 0]  CenterOfMassUnits=m  MomentsOfInertia=[1 1 1]  MomentsOfInertiaUnits=kg*m^2  ProductsOfInertia=[0 0 0]  ProductsOfInertiaUnits=kg*m^2  DensityBased=on  Density=1000  DensityUnits=kg/(m^3)  DoExposeReferenceFrame=on  SerializedFrames=<Frames/>  GraphicType=FromGeometry  MarkerShape=Sphere  MarkerSize=10  MarkerSizeUnits=m  GraphicVisPropType=SimpleVisualProperties  GraphicDiffuseColor=[0.5 0.5 0.5]  GraphicSpecularColor=[0.5 0.5 0.5 1.0]  GraphicAmbientColor=[0.15 0.15 0.15 1.0]  GraphicEmissiveColor=[0.0 0.0 0.0 1.0]  GraphicShininess=75  GraphicOpacity=1.0  GeometryShape=Brick  RectangleSize=[1 1]  RectangleSizeUnits=m  BrickDimensions=[table.l table.w table.h]  BrickDimensionUnits=m  CylinderRadius=1  CylinderRadiusUnits=m  CylinderLength=1  CylinderLengthUnits=m  SphereRadius=1  SphereRadiusUnits=m  EllipsoidRadii=[1 1 1]  EllipsoidRadiiUnits=m  ExtrusionCrossSection=[1 1; -1 1; -1 -1; 1 -1]  ExtrusionCrossSectionUnits=m  ExtrusionLength=1  ExtrusionLengthUnits=m  PolygonNumSides=3  PolygonOuterRadius=1  PolygonOuterRadiusUnits=m  ExtGeomFileType=STL  ExtGeomFileUnits=m  RevolutionCrossSection=[1 1; 1 -1; 2 -1; 2 1]  RevolutionCrossSectionUnits=m  RevolutionExtent=Full  RevolutionAngle=180  RevolutionAngleUnits=deg
  Transform Contact Ref : sm_lib/Frames and Transforms/Rigid Transform  TranslationMethod=None  TranslationLengthUnit=m  TranslationStandardAxis=+X  TranslationStandardOffset=3/2  TranslationCartesianOffset=[1 0 -1]  TranslationROffset=0  TranslationROffsetUnits=m  TranslationZOffset=0  TranslationZOffsetUnits=m  TranslationThetaOffset=0  TranslationThetaOffsetUnits=deg  RotationMethod=StandardAxis  RotationAngleUnits=deg  RotationStandardAxis=+Z  RotationAngle=90  RotationArbitraryAxis=[0 0 1]  FollAlignAxisA=+X  BaseAlignAxisA=+Y  FollAlignAxisB=+Y  BaseAlignAxisB=+Z  RotationSequenceAxes=FollowerAxes  RotationSequence=XYX  RotationSequenceAngles=[0 0 0]  RotationSequenceAnglesUnits=deg  RotationMatrix=[1 0 0; 0 1 0; 0 0 1]
  Transform Contact Ref1 : sm_lib/Frames and Transforms/Rigid Transform  TranslationMethod=Cartesian  TranslationLengthUnit=m  TranslationStandardAxis=+X  TranslationStandardOffset=3/2  TranslationCartesianOffset=[0 ground_y 0]  TranslationROffset=0  TranslationROffsetUnits=m  TranslationZOffset=0  TranslationZOffsetUnits=m  TranslationThetaOffset=0  TranslationThetaOffsetUnits=deg  RotationMethod=None  RotationAngleUnits=deg  RotationStandardAxis=+Z  RotationAngle=90  RotationArbitraryAxis=[0 0 1]  FollAlignAxisA=+X  BaseAlignAxisA=+Y  FollAlignAxisB=+Y  BaseAlignAxisB=+Z  RotationSequenceAxes=FollowerAxes  RotationSequence=XYX  RotationSequenceAngles=[0 0 0]  RotationSequenceAnglesUnits=deg  RotationMatrix=[1 0 0; 0 1 0; 0 0 1]
  F : PMIOPort  Port=1  Side=Right
  B : PMIOPort  Port=2  Side=Left
  connections:
  Transform Contact Ref/LConn1 -- Transform Contact Ref1/RConn1 -- Solid/RConn1
  Transform Contact Ref/RConn1 -- F/RConn1
  B/RConn1 -- Transform Contact Ref1/LConn1

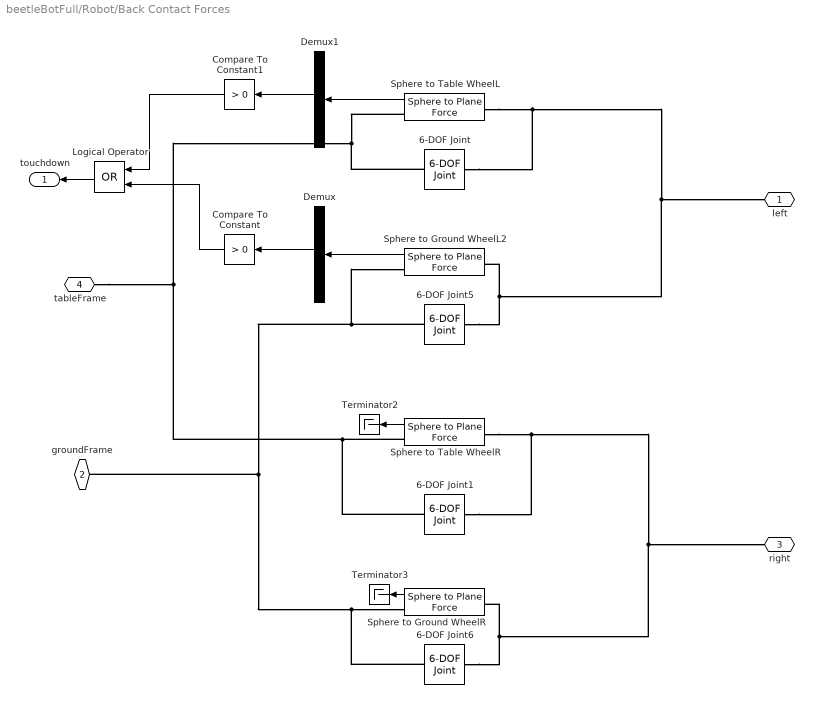
== system beetleBotFull/Robot/Back Contact Forces ==
  6-DOF Joint{,1,5..6} (4 alike) : sm_lib/Joints/6-DOF Joint  SenseConstraintForce=off  SenseConstraintForceX=off  SenseConstraintForceY=off  SenseConstraintForceZ=off  SenseConstraintTorque=off  SenseConstraintTorqueX=off  SenseConstraintTorqueY=off  SenseConstraintTorqueZ=off  SenseTotalForce=off  SenseTotalForceX=off  SenseTotalForceY=off  SenseTotalForceZ=off  SenseTotalTorque=off  SenseTotalTorqueX=off  SenseTotalTorqueY=off  SenseTotalTorqueZ=off  CompositeWrenchDir=FollowerOnBase  CompositeWrenchFrame=BaseFrame  PxEquilibriumPosition=0  PxEquilibriumPositionUnits=m  PxSpringStiffness=0  PxSpringStiffnessUnits=N/m  PxDampingCoefficient=0  PxDampingCoefficientUnits=N/(m/s)  PxTorqueActuationMode=NoTorque  PxMotionActuationMode=ComputedMotion  PxSensePosition=off  PxSenseVelocity=off  PxSenseAcceleration=off  PxSenseTorqueForce=off  PxPositionTargetSpecify=off  PxPositionTargetPriority=High  PxPositionTargetValue=0  PxPositionTargetValueUnits=m  PxVelocityTargetSpecify=off  PxVelocityTargetPriority=High  PxVelocityTargetValue=0  PxVelocityTargetValueUnits=m/s  PyEquilibriumPosition=0  PyEquilibriumPositionUnits=m  PySpringStiffness=0  PySpringStiffnessUnits=N/m  PyDampingCoefficient=0  PyDampingCoefficientUnits=N/(m/s)  PyTorqueActuationMode=NoTorque  PyMotionActuationMode=ComputedMotion  PySensePosition=off  PySenseVelocity=off  PySenseAcceleration=off  PySenseTorqueForce=off  PyPositionTargetSpecify=off  PyPositionTargetPriority=High  PyPositionTargetValue=0  PyPositionTargetValueUnits=m  PyVelocityTargetSpecify=off  PyVelocityTargetPriority=High  PyVelocityTargetValue=0  PyVelocityTargetValueUnits=m/s  PzEquilibriumPosition=0  PzEquilibriumPositionUnits=m  PzSpringStiffness=0  PzSpringStiffnessUnits=N/m  PzDampingCoefficient=0  PzDampingCoefficientUnits=N/(m/s)  PzTorqueActuationMode=NoTorque  PzMotionActuationMode=ComputedMotion  PzSensePosition=off  PzSenseVelocity=off  PzSenseAcceleration=off  PzSenseTorqueForce=off  PzPositionTargetSpecify=off  PzPositionTargetPriority=High  PzPositionTargetValue=2  PzPositionTargetValueUnits=m  PzVelocityTargetSpecify=off  PzVelocityTargetPriority=High  PzVelocityTargetValue=0  PzVelocityTargetValueUnits=m/s  SphDefPosRotationMethod=None  SphDefPosRotationAngleUnits=deg  SphDefPosRotationStandardAxis=+Z  SphDefPosRotationAngle=0.0  SphDefPosRotationArbitraryAxis=[0 0 1]  SphDefPosFollAlignAxisA=+X  SphDefPosBaseAlignAxisA=+Y  SphDefPosFollAlignAxisB=+Y  SphDefPosBaseAlignAxisB=+Z  SphDefPosRotationSequenceAxes=FollowerAxes  SphDefPosRotationSequence=XYX  SphDefPosRotationSequenceAngles=[0 0 0]  SphDefPosRotationSequenceAnglesUnits=deg  SphDefPosRotationMatrix=[1 0 0; 0 1 0; 0 0 1]  SphEqPosRotationMethod=None  SphEqPosRotationAngleUnits=deg  SphEqPosRotationStandardAxis=+Z  SphEqPosRotationAngle=0.0  SphEqPosRotationArbitraryAxis=[0 0 1]  SphEqPosFollAlignAxisA=+X  SphEqPosBaseAlignAxisA=+Y  SphEqPosFollAlignAxisB=+Y  SphEqPosBaseAlignAxisB=+Z  SphEqPosRotationSequenceAxes=FollowerAxes  SphEqPosRotationSequence=XYX  SphEqPosRotationSequenceAngles=[0 0 0]  SphEqPosRotationSequenceAnglesUnits=deg  SphEqPosRotationMatrix=[1 0 0; 0 1 0; 0 0 1]  SphSpringStiffness=0  SphSpringStiffnessUnits=N*m/deg  SphDampingCoefficient=0  SphDampingCoefficientUnits=N*m/(deg/s)  SphActuateTorqueX=off  SphActuateTorqueY=off  SphActuateTorqueZ=off  SphActuateTorque=off  SphTorqueActuationMode=NoTorque  SphMotionActuationMode=ComputedMotion  SphActuationFrame=BaseFrame  SphSensePosition=off  SphSenseVelocityX=off  SphSenseVelocityY=off  SphSenseVelocityZ=off  SphSenseVelocity=off  SphSenseAccelerationX=off  SphSenseAccelerationY=off  SphSenseAccelerationZ=off  SphSenseAcceleration=off  SphSenseTorqueX=off  SphSenseTorqueY=off  SphSenseTorqueZ=off  SphSenseTorqueForce=off  SphSensingFrame=BaseFrame  SphPositionTargetRotationMethod=None  SphPositionTargetRotationAngleUnits=deg  SphPositionTargetRotationStandardAxis=+Z  SphPositionTargetRotationAngle=0.0  SphPositionTargetRotationArbitraryAxis=[0 0 1]  SphPositionTargetFollAlignAxisA=+X  SphPositionTargetBaseAlignAxisA=+Y  SphPositionTargetFollAlignAxisB=+Y  SphPositionTargetBaseAlignAxisB=+Z  SphPositionTargetRotationSequenceAxes=FollowerAxes  SphPositionTargetRotationSequence=XYX  SphPositionTargetRotationSequenceAngles=[0 0 0]  SphPositionTargetRotationSequenceAnglesUnits=deg  SphPositionTargetRotationMatrix=[1 0 0; 0 1 0; 0 0 1]  SphPositionTargetSpecify=off  SphPositionTargetPriority=High  SphVelocityTargetValue=[0 0 0]  SphVelocityTargetValueUnits=deg/s  SphVelocityTargetSpecify=off  SphVelocityTargetPriority=High  SphVelocityTargetInFollowerFrame=on
  Compare To Constant : simulink/Logic and Bit Operations/Compare To Constant  relop=>  const=0  OutDataTypeStr=boolean
  Compare To Constant1 : simulink/Logic and Bit Operations/Compare To Constant  relop=>  const=0  OutDataTypeStr=boolean
  Demux : Demux  Outputs=8
  Demux1 : Demux  Outputs=8
  Logical Operator : Logic  Operator=OR  AllPortsSameDT=off  OutDataTypeStr=boolean
  Sphere to Ground WheelL2 : Contact_Forces_Lib/3D/Sphere to Plane Force  sphere_rad=3*0.0254  plane_lenx=table.l  plane_leny=table.w  plane_depth=table.h/2  force_law=Linear  k_contact=1e5  b_contact=1e4  pen_full_damp_F=1e-4  pen_exponent=1  custom_param_1=1  custom_param_2=1  friction_law=Stick-Slip Continuous  mu_kinetic=kinetic_friction  mu_static=static_friction  v_thr=0.005  vis_on=off  vis_opc_en=0  vis_len_plaBz=table.h*0.1  vis_clr=[0.9 0.2 0.2]  vis_opc=0.7
  Sphere to Ground WheelR : Contact_Forces_Lib/3D/Sphere to Plane Force  sphere_rad=3*0.0254  plane_lenx=table.l  plane_leny=table.w  plane_depth=table.h/2  force_law=Linear  k_contact=1e5  b_contact=1e4  pen_full_damp_F=1e-4  pen_exponent=1  custom_param_1=1  custom_param_2=1  friction_law=Stick-Slip Continuous  mu_kinetic=kinetic_friction  mu_static=static_friction  v_thr=0.005  vis_on=off  vis_opc_en=0  vis_len_plaBz=table.h*0.1  vis_clr=[0.9 0.2 0.2]  vis_opc=0.7
  Sphere to Table WheelL : Contact_Forces_Lib/3D/Sphere to Plane Force  sphere_rad=3*0.0254  plane_lenx=table.l  plane_leny=table.w  plane_depth=table.h/2  force_law=Linear  k_contact=1e5  b_contact=1e4  pen_full_damp_F=1e-4  pen_exponent=1  custom_param_1=1  custom_param_2=1  friction_law=Stick-Slip Continuous  mu_kinetic=kinetic_friction  mu_static=static_friction  v_thr=0.005  vis_on=off  vis_opc_en=0  vis_len_plaBz=table.h*0.1  vis_clr=[0.9 0.2 0.2]  vis_opc=0.7
  Sphere to Table WheelR : Contact_Forces_Lib/3D/Sphere to Plane Force  sphere_rad=3*0.0254  plane_lenx=table.l  plane_leny=table.w  plane_depth=table.h/2  force_law=Linear  k_contact=1e5  b_contact=1e4  pen_full_damp_F=1e-4  pen_exponent=1  custom_param_1=1  custom_param_2=1  friction_law=Stick-Slip Continuous  mu_kinetic=kinetic_friction  mu_static=static_friction  v_thr=0.005  vis_on=off  vis_opc_en=0  vis_len_plaBz=table.h*0.1  vis_clr=[0.9 0.2 0.2]  vis_opc=0.7
  Terminator2 : Terminator
  Terminator3 : Terminator
  left : PMIOPort  Port=1  Side=Right
  groundFrame : PMIOPort  Port=2  Side=Left
  right : PMIOPort  Port=3  Side=Right
  tableFrame : PMIOPort  Port=4  Side=Left
  touchdown : Outport
  wires:
  Sphere to Table WheelR/1 -> Terminator2/1
  Sphere to Table WheelL/1 -> Demux1/1
  Sphere to Ground WheelR/1 -> Terminator3/1
  Sphere to Ground WheelL2/1 -> Demux/1
  Demux/4 -> Compare To Constant/1
  Compare To Constant/1 -> Logical Operator/2
  Demux1/4 -> Compare To Constant1/1
  Compare To Constant1/1 -> Logical Operator/1
  Logical Operator/1 -> touchdown/1
  connections:
  Sphere to Table WheelR/RConn1 -- Sphere to Table WheelL/RConn1 -- 6-DOF Joint/LConn1 -- tableFrame/RConn1 -- 6-DOF Joint1/LConn1
  6-DOF Joint6/LConn1 -- 6-DOF Joint5/LConn1 -- Sphere to Ground WheelL2/RConn1 -- groundFrame/RConn1 -- Sphere to Ground WheelR/RConn1
  6-DOF Joint5/RConn1 -- 6-DOF Joint/RConn1 -- Sphere to Table WheelL/LConn1 -- left/RConn1 -- Sphere to Ground WheelL2/LConn1
  6-DOF Joint6/RConn1 -- Sphere to Table WheelR/LConn1 -- 6-DOF Joint1/RConn1 -- right/RConn1 -- Sphere to Ground WheelR/LConn1

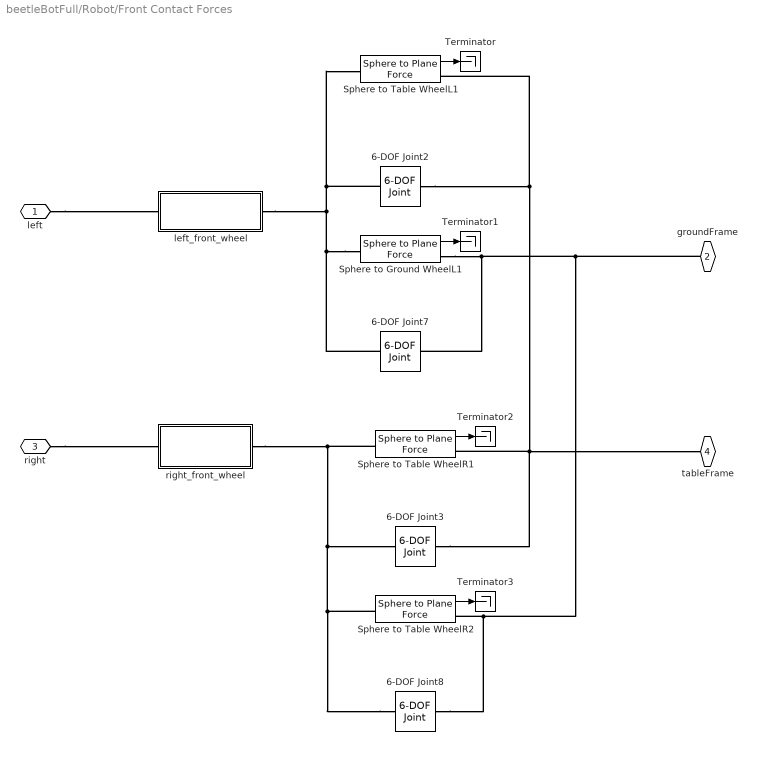
== system beetleBotFull/Robot/Front Contact Forces ==
  6-DOF Joint{2..3,7..8} (4 alike) : sm_lib/Joints/6-DOF Joint  SenseConstraintForce=off  SenseConstraintForceX=off  SenseConstraintForceY=off  SenseConstraintForceZ=off  SenseConstraintTorque=off  SenseConstraintTorqueX=off  SenseConstraintTorqueY=off  SenseConstraintTorqueZ=off  SenseTotalForce=off  SenseTotalForceX=off  SenseTotalForceY=off  SenseTotalForceZ=off  SenseTotalTorque=off  SenseTotalTorqueX=off  SenseTotalTorqueY=off  SenseTotalTorqueZ=off  CompositeWrenchDir=FollowerOnBase  CompositeWrenchFrame=BaseFrame  PxEquilibriumPosition=0  PxEquilibriumPositionUnits=m  PxSpringStiffness=0  PxSpringStiffnessUnits=N/m  PxDampingCoefficient=0  PxDampingCoefficientUnits=N/(m/s)  PxTorqueActuationMode=NoTorque  PxMotionActuationMode=ComputedMotion  PxSensePosition=off  PxSenseVelocity=off  PxSenseAcceleration=off  PxSenseTorqueForce=off  PxPositionTargetSpecify=off  PxPositionTargetPriority=High  PxPositionTargetValue=0  PxPositionTargetValueUnits=m  PxVelocityTargetSpecify=off  PxVelocityTargetPriority=High  PxVelocityTargetValue=0  PxVelocityTargetValueUnits=m/s  PyEquilibriumPosition=0  PyEquilibriumPositionUnits=m  PySpringStiffness=0  PySpringStiffnessUnits=N/m  PyDampingCoefficient=0  PyDampingCoefficientUnits=N/(m/s)  PyTorqueActuationMode=NoTorque  PyMotionActuationMode=ComputedMotion  PySensePosition=off  PySenseVelocity=off  PySenseAcceleration=off  PySenseTorqueForce=off  PyPositionTargetSpecify=off  PyPositionTargetPriority=High  PyPositionTargetValue=0  PyPositionTargetValueUnits=m  PyVelocityTargetSpecify=off  PyVelocityTargetPriority=High  PyVelocityTargetValue=0  PyVelocityTargetValueUnits=m/s  PzEquilibriumPosition=0  PzEquilibriumPositionUnits=m  PzSpringStiffness=0  PzSpringStiffnessUnits=N/m  PzDampingCoefficient=0  PzDampingCoefficientUnits=N/(m/s)  PzTorqueActuationMode=NoTorque  PzMotionActuationMode=ComputedMotion  PzSensePosition=off  PzSenseVelocity=off  PzSenseAcceleration=off  PzSenseTorqueForce=off  PzPositionTargetSpecify=off  PzPositionTargetPriority=High  PzPositionTargetValue=2  PzPositionTargetValueUnits=m  PzVelocityTargetSpecify=off  PzVelocityTargetPriority=High  PzVelocityTargetValue=0  PzVelocityTargetValueUnits=m/s  SphDefPosRotationMethod=None  SphDefPosRotationAngleUnits=deg  SphDefPosRotationStandardAxis=+Z  SphDefPosRotationAngle=0.0  SphDefPosRotationArbitraryAxis=[0 0 1]  SphDefPosFollAlignAxisA=+X  SphDefPosBaseAlignAxisA=+Y  SphDefPosFollAlignAxisB=+Y  SphDefPosBaseAlignAxisB=+Z  SphDefPosRotationSequenceAxes=FollowerAxes  SphDefPosRotationSequence=XYX  SphDefPosRotationSequenceAngles=[0 0 0]  SphDefPosRotationSequenceAnglesUnits=deg  SphDefPosRotationMatrix=[1 0 0; 0 1 0; 0 0 1]  SphEqPosRotationMethod=None  SphEqPosRotationAngleUnits=deg  SphEqPosRotationStandardAxis=+Z  SphEqPosRotationAngle=0.0  SphEqPosRotationArbitraryAxis=[0 0 1]  SphEqPosFollAlignAxisA=+X  SphEqPosBaseAlignAxisA=+Y  SphEqPosFollAlignAxisB=+Y  SphEqPosBaseAlignAxisB=+Z  SphEqPosRotationSequenceAxes=FollowerAxes  SphEqPosRotationSequence=XYX  SphEqPosRotationSequenceAngles=[0 0 0]  SphEqPosRotationSequenceAnglesUnits=deg  SphEqPosRotationMatrix=[1 0 0; 0 1 0; 0 0 1]  SphSpringStiffness=0  SphSpringStiffnessUnits=N*m/deg  SphDampingCoefficient=0  SphDampingCoefficientUnits=N*m/(deg/s)  SphActuateTorqueX=off  SphActuateTorqueY=off  SphActuateTorqueZ=off  SphActuateTorque=off  SphTorqueActuationMode=NoTorque  SphMotionActuationMode=ComputedMotion  SphActuationFrame=BaseFrame  SphSensePosition=off  SphSenseVelocityX=off  SphSenseVelocityY=off  SphSenseVelocityZ=off  SphSenseVelocity=off  SphSenseAccelerationX=off  SphSenseAccelerationY=off  SphSenseAccelerationZ=off  SphSenseAcceleration=off  SphSenseTorqueX=off  SphSenseTorqueY=off  SphSenseTorqueZ=off  SphSenseTorqueForce=off  SphSensingFrame=BaseFrame  SphPositionTargetRotationMethod=None  SphPositionTargetRotationAngleUnits=deg  SphPositionTargetRotationStandardAxis=+Z  SphPositionTargetRotationAngle=0.0  SphPositionTargetRotationArbitraryAxis=[0 0 1]  SphPositionTargetFollAlignAxisA=+X  SphPositionTargetBaseAlignAxisA=+Y  SphPositionTargetFollAlignAxisB=+Y  SphPositionTargetBaseAlignAxisB=+Z  SphPositionTargetRotationSequenceAxes=FollowerAxes  SphPositionTargetRotationSequence=XYX  SphPositionTargetRotationSequenceAngles=[0 0 0]  SphPositionTargetRotationSequenceAnglesUnits=deg  SphPositionTargetRotationMatrix=[1 0 0; 0 1 0; 0 0 1]  SphPositionTargetSpecify=off  SphPositionTargetPriority=High  SphVelocityTargetValue=[0 0 0]  SphVelocityTargetValueUnits=deg/s  SphVelocityTargetSpecify=off  SphVelocityTargetPriority=High  SphVelocityTargetInFollowerFrame=on
  Sphere to Ground WheelL1 : Contact_Forces_Lib/3D/Sphere to Plane Force  sphere_rad=3*0.0254  plane_lenx=table.l  plane_leny=table.w  plane_depth=table.h/2  force_law=Linear  k_contact=1e5  b_contact=1e4  pen_full_damp_F=1e-4  pen_exponent=1  custom_param_1=1  custom_param_2=1  friction_law=Stick-Slip Continuous  mu_kinetic=0.5  mu_static=0.8  v_thr=0.005  vis_on=off  vis_opc_en=0  vis_len_plaBz=table.h*0.1  vis_clr=[0.9 0.2 0.2]  vis_opc=0.7
  Sphere to Table WheelL1 : Contact_Forces_Lib/3D/Sphere to Plane Force  sphere_rad=3*0.0254  plane_lenx=table.l  plane_leny=table.w  plane_depth=table.h/2  force_law=Linear  k_contact=1e5  b_contact=1e4  pen_full_damp_F=1e-4  pen_exponent=1  custom_param_1=1  custom_param_2=1  friction_law=Stick-Slip Continuous  mu_kinetic=0.5  mu_static=0.8  v_thr=0.005  vis_on=off  vis_opc_en=0  vis_len_plaBz=table.h*0.1  vis_clr=[0.9 0.2 0.2]  vis_opc=0.7
  Sphere to Table WheelR1 : Contact_Forces_Lib/3D/Sphere to Plane Force  sphere_rad=3*0.0254  plane_lenx=table.l  plane_leny=table.w  plane_depth=table.h/2  force_law=Linear  k_contact=1e5  b_contact=1e4  pen_full_damp_F=1e-4  pen_exponent=1  custom_param_1=1  custom_param_2=1  friction_law=Stick-Slip Continuous  mu_kinetic=0.5  mu_static=0.8  v_thr=0.005  vis_on=off  vis_opc_en=0  vis_len_plaBz=table.h*0.1  vis_clr=[0.9 0.2 0.2]  vis_opc=0.7
  Sphere to Table WheelR2 : Contact_Forces_Lib/3D/Sphere to Plane Force  sphere_rad=3*0.0254  plane_lenx=table.l  plane_leny=table.w  plane_depth=table.h/2  force_law=Linear  k_contact=1e5  b_contact=1e4  pen_full_damp_F=1e-4  pen_exponent=1  custom_param_1=1  custom_param_2=1  friction_law=Stick-Slip Continuous  mu_kinetic=0.5  mu_static=0.8  v_thr=0.005  vis_on=off  vis_opc_en=0  vis_len_plaBz=table.h*0.1  vis_clr=[0.9 0.2 0.2]  vis_opc=0.7
  Terminator{,1..3} (4 alike) : Terminator
  left_front_wheel : Subsystem
  right_front_wheel : Subsystem
  left : PMIOPort  Port=1  Side=Left
  groundFrame : PMIOPort  Port=2  Side=Right
  right : PMIOPort  Port=3  Side=Left
  tableFrame : PMIOPort  Port=4  Side=Right
  wires:
  Sphere to Table WheelR1/1 -> Terminator2/1
  Sphere to Table WheelR2/1 -> Terminator3/1
  Sphere to Table WheelL1/1 -> Terminator/1
  Sphere to Ground WheelL1/1 -> Terminator1/1
  connections:
  Sphere to Ground WheelL1/RConn1 -- Sphere to Table WheelR2/RConn1 -- 6-DOF Joint8/RConn1 -- groundFrame/RConn1 -- 6-DOF Joint7/RConn1
  Sphere to Ground WheelL1/LConn1 -- Sphere to Table WheelL1/LConn1 -- 6-DOF Joint2/LConn1 -- left_front_wheel/RConn1 -- 6-DOF Joint7/LConn1
  Sphere to Table WheelR1/RConn1 -- 6-DOF Joint3/RConn1 -- tableFrame/RConn1 -- 6-DOF Joint2/RConn1 -- Sphere to Table WheelL1/RConn1
  6-DOF Joint8/LConn1 -- 6-DOF Joint3/LConn1 -- Sphere to Table WheelR1/LConn1 -- right_front_wheel/RConn1 -- Sphere to Table WheelR2/LConn1
  right/RConn1 -- right_front_wheel/LConn1
  left/RConn1 -- left_front_wheel/LConn1

== system beetleBotFull/Robot/battery ==
  ReferenceFrame : sm_lib/Frames and Transforms/Reference Frame
  Solid : sm_lib/Body Elements/Solid  InertiaType=Custom  Mass=smiData.Solid(6).mass  MassUnits=kg  CenterOfMass=smiData.Solid(6).CoM  CenterOfMassUnits=mm  MomentsOfInertia=smiData.Solid(6).MoI  MomentsOfInertiaUnits=kg*mm^2  ProductsOfInertia=smiData.Solid(6).PoI  ProductsOfInertiaUnits=kg*mm^2  DensityBased=on  Density=1000  DensityUnits=kg/(m^3)  DoExposeReferenceFrame=on  SerializedFrames=<Frames/>  GraphicType=FromGeometry  MarkerShape=Sphere  MarkerSize=10  GraphicVisPropType=SimpleVisualProperties  GraphicDiffuseColor=smiData.Solid(6).color  GraphicSpecularColor=[0.5 0.5 0.5 1.0]  GraphicAmbientColor=[0.15 0.15 0.15 1.0]  GraphicEmissiveColor=[0.0 0.0 0.0 1.0]  GraphicShininess=75  GraphicOpacity=smiData.Solid(6).opacity  GeometryShape=FromFile  RectangleSize=[1 1]  RectangleSizeUnits=m  BrickDimensions=[1 1 1]  BrickDimensionUnits=m  CylinderRadius=1  CylinderRadiusUnits=m  CylinderLength=1  CylinderLengthUnits=m  SphereRadius=1  SphereRadiusUnits=m  EllipsoidRadii=[1 1 1]  EllipsoidRadiiUnits=m  ExtrusionCrossSection=[1 1; -1 1; -1 -1; 1 -1]  ExtrusionCrossSectionUnits=m  ExtrusionLength=1  ExtrusionLengthUnits=m  PolygonNumSides=3  PolygonOuterRadius=1  PolygonOuterRadiusUnits=m  ExtGeomFileType=STEP  ExtGeomFileName=battery mockup_Default_sldprt.STEP  ExtGeomFileUnits=m  RevolutionCrossSection=[1 1; 1 -1; 2 -1; 2 1]  RevolutionCrossSectionUnits=m  RevolutionExtent=Full  RevolutionAngle=180  RevolutionAngleUnits=deg
  Transform : sm_lib/Frames and Transforms/Rigid Transform  TranslationMethod=Cartesian  TranslationLengthUnit=mm  TranslationStandardAxis=+Z  TranslationStandardOffset=0  TranslationCartesianOffset=smiData.RigidTransform(14).translation  TranslationROffset=0  TranslationROffsetUnits=m  TranslationZOffset=0  TranslationZOffsetUnits=m  TranslationThetaOffset=0  TranslationThetaOffsetUnits=deg  RotationMethod=ArbitraryAxis  RotationAngleUnits=rad  RotationStandardAxis=+Z  RotationAngle=smiData.RigidTransform(14).angle  RotationArbitraryAxis=smiData.RigidTransform(14).axis  FollAlignAxisA=+X  BaseAlignAxisA=+Y  FollAlignAxisB=+Y  BaseAlignAxisB=+Z  RotationSequenceAxes=FollowerAxes  RotationSequence=XYX  RotationSequenceAngles=[0 0 0]  RotationSequenceAnglesUnits=deg  RotationMatrix=[1 0 0; 0 1 0; 0 0 1]
  F : PMIOPort  Port=1  Side=Left
  connections:
  Solid/RConn1 -- ReferenceFrame/RConn1 -- Transform/LConn1
  Transform/RConn1 -- F/RConn1
